simulink model "vnsimulink"  (R2020a)
settings: Solver=ode4  StartTime=0.0  StopTime=20  FixedStep=8e-6  RelTol=1e-3
undefined symbols (not defined in the file or in its folder): D1, Delta, sigbuilder_block
libraries: powerlib x98, powerlib_meascontrol x21, simulink x16
(part 2 of 3)

== system vnsimulink/PV15kW1/Subsystem2 ==
  Current : powerlib/Measurements/Current Measurement  PhasorSimulation=off  OutputType=Complex  PSBequivalent=0
  Current 2 : powerlib/Measurements/Current Measurement  PhasorSimulation=off  OutputType=Complex  PSBequivalent=0
  Current1 : powerlib/Measurements/Current Measurement  PhasorSimulation=off  OutputType=Complex  PSBequivalent=0
  1 : PMIOPort  Side=Left
  2 : PMIOPort  Port=2  Side=Right
  3 : PMIOPort  Port=3  Side=Left
  4 : PMIOPort  Port=4  Side=Right
  5 : PMIOPort  Port=5  Side=Left
  6 : PMIOPort  Port=6  Side=Right
  O1 : Outport
  O2 : Outport  Port=2
  O3 : Outport  Port=3
  wires:
  Current 2/1 -> O3/1
  Current1/1 -> O2/1
  Current/1 -> O1/1
  connections:
  6/RConn1 -- Current 2/RConn1
  5/RConn1 -- Current 2/LConn1
  4/RConn1 -- Current1/RConn1
  3/RConn1 -- Current1/LConn1
  2/RConn1 -- Current/RConn1
  1/RConn1 -- Current/LConn1

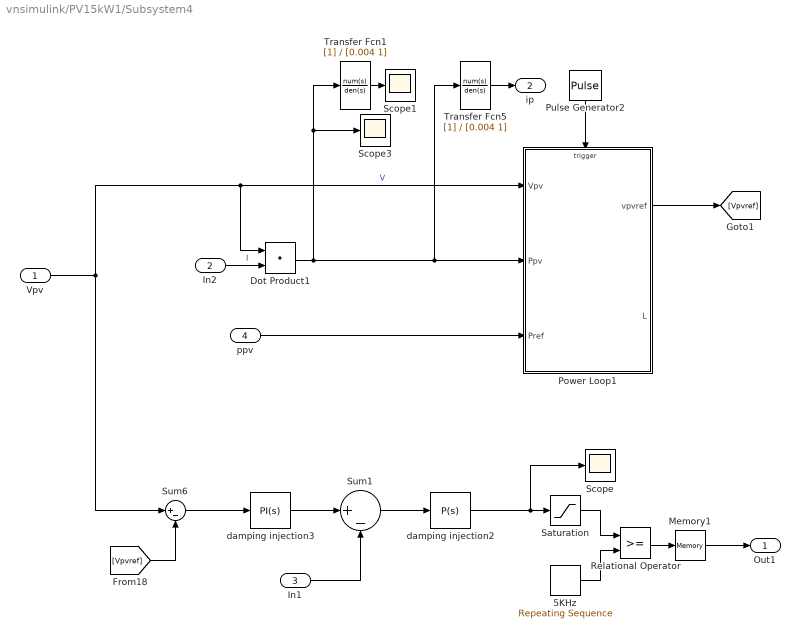
== system vnsimulink/PV15kW1/Subsystem4 ==
  Vpv : Inport
  In2 : Inport  Port=2
  In1 : Inport  Port=3
  ppv : Inport  Port=4
  5KHz : simulink/Sources/Repeating Sequence  rep_seq_t=[0 1e-4 2e-4]  rep_seq_y=[0 1 0]
  Dot Product1 : DotProduct  InputSameDT=on  OutDataTypeStr=Inherit: Inherit via internal rule
  Memory1 : Memory
  Power Loop1 : Subsystem  TreatAsAtomicUnit=on
  Pulse Generator2 : DiscretePulseGenerator  PulseType=Time based  Period=20e-4  PulseWidth=50
  Relational Operator : RelationalOperator  OutDataTypeStr=boolean  RndMeth=Nearest
  Saturation : Saturate  UpperLimit=0.9  LowerLimit=0
  Scope : Scope
  Scope1 : Scope
  Scope3 : Scope
  Sum1 : Sum  Inputs=|+-
  Sum6 : Sum  Inputs=|+-
  Transfer Fcn1 : TransferFcn  Denominator=[0.004 1]
  Transfer Fcn5 : TransferFcn  Denominator=[0.004 1]
  damping injection2 : simulink/Continuous/PID Controller  Controller=P  Form=Parallel  TimeDomain=Continuous-time  UseExternalTs=off  SampleTime=1  IntegratorMethod=Forward Euler  FilterMethod=Forward Euler  ControllerParametersSource=internal  P=0.015  I=0.15  D=0  UseFilter=on  N=100  TunerSelectOption=Transfer Function Based (PID Tuner App)  InitialConditionSource=internal  InitialConditionForIntegrator=0  InitialConditionForFilter=0  DifferentiatorICPrevScaledInput=0  ExternalReset=none  TrackingMode=off  Kt=1  LimitOutput=off  UpperSaturationLimit=inf  LowerSaturationLimit=-inf  LinearizeAsGain=on  AntiWindupMode=none  Kb=1  POutMin=[]  POutMax=[]  IOutMin=[]  IOutMax=[]  DOutMin=[]  DOutMax=[]  NOutMin=[]  NOutMax=[]  SumOutMin=[]  SumOutMax=[]  SaturationOutMin=[]  SaturationOutMax=[]  PParamMin=[]  PParamMax=[]  IParamMin=[]  IParamMax=[]  DParamMin=[]  DParamMax=[]  NParamMin=[]  NParamMax=[]  KbParamMin=[]  KbParamMax=[]  KtParamMin=[]  KtParamMax=[]  KbOutMin=[]  KbOutMax=[]  KtOutMin=[]  KtOutMax=[]  IntegratorOutMin=[]  IntegratorOutMax=[]  FilterOutMin=[]  FilterOutMax=[]  SumI1OutMin=[]  SumI1OutMax=[]  SumI2OutMin=[]  SumI2OutMax=[]  SumI3OutMin=[]  SumI3OutMax=[]  SumI4OutMin=[]  SumI4OutMax=[]  SumDOutMin=[]  SumDOutMax=[]  DifferentiatorOutMin=[]  DifferentiatorOutMax=[]  FilterDiffOutCoefMin=[]  FilterDiffOutCoefMax=[]  ReciprocalOutMin=[]  ReciprocalOutMax=[]  SumDenOutMin=[]  SumDenOutMax=[]  SumNumOutMin=[]  SumNumOutMax=[]  DivideOutMin=[]  DivideOutMax=[]  UdiffTsProdOutMin=[]  UdiffTsProdOutMax=[]  NTsProdOutMin=[]  NTsProdOutMax=[]  UintegralTsProdOutMin=[]  UintegralTsProdOutMax=[]  UngainTsProdOutMin=[]  UngainTsProdOutMax=[]  IntegratorContinuousStateAttributes=''  IntegratorStateMustResolveToSignalObject=off  IntegratorRTWStateStorageClass=Auto  FilterContinuousStateAttributes=''  FilterStateMustResolveToSignalObject=off  FilterRTWStateStorageClass=Auto  ParallelPVariant=InternalParameters  IdealPVariant=Disabled  IVariant=Disabled  DVariant=Disabled  IntegratorVariant=Disabled  SatVariant=Disabled  AWVariant=Disabled  PCopyVariant=Disabled  TRVariant=Disabled  FdbkBlocksVariant=Forward  IdealPFdbkVariant=Disabled  SatFdbkVariant=Disabled  DerivativeFilterVariant=Disabled  NVariant=Disabled  NCopyVariant=Disabled_SignalSpec  FilterICVariant=Disabled  IntegratorICVariant=Disabled  ExternalResetVariant=Disabled  TRSumVariant=Passthrough  SumFdbkVariant=Disabled  SumVariant=Passthrough_P  TsampFilterVariant=InternalTs  TsampNgainVariant=Passthrough  TsampIntegralVariant=Disabled_SignalSpec
  damping injection3 : simulink/Continuous/PID Controller  Controller=PI  Form=Parallel  TimeDomain=Continuous-time  UseExternalTs=off  SampleTime=1  IntegratorMethod=Forward Euler  FilterMethod=Forward Euler  ControllerParametersSource=internal  P=0.3  I=6  D=0  UseFilter=on  N=100  TunerSelectOption=Transfer Function Based (PID Tuner App)  InitialConditionSource=internal  InitialConditionForIntegrator=0  InitialConditionForFilter=0  DifferentiatorICPrevScaledInput=0  ExternalReset=none  TrackingMode=off  Kt=1  LimitOutput=off  UpperSaturationLimit=inf  LowerSaturationLimit=-inf  LinearizeAsGain=on  AntiWindupMode=none  Kb=1  POutMin=[]  POutMax=[]  IOutMin=[]  IOutMax=[]  DOutMin=[]  DOutMax=[]  NOutMin=[]  NOutMax=[]  SumOutMin=[]  SumOutMax=[]  SaturationOutMin=[]  SaturationOutMax=[]  PParamMin=[]  PParamMax=[]  IParamMin=[]  IParamMax=[]  DParamMin=[]  DParamMax=[]  NParamMin=[]  NParamMax=[]  KbParamMin=[]  KbParamMax=[]  KtParamMin=[]  KtParamMax=[]  KbOutMin=[]  KbOutMax=[]  KtOutMin=[]  KtOutMax=[]  IntegratorOutMin=[]  IntegratorOutMax=[]  FilterOutMin=[]  FilterOutMax=[]  SumI1OutMin=[]  SumI1OutMax=[]  SumI2OutMin=[]  SumI2OutMax=[]  SumI3OutMin=[]  SumI3OutMax=[]  SumI4OutMin=[]  SumI4OutMax=[]  SumDOutMin=[]  SumDOutMax=[]  DifferentiatorOutMin=[]  DifferentiatorOutMax=[]  FilterDiffOutCoefMin=[]  FilterDiffOutCoefMax=[]  ReciprocalOutMin=[]  ReciprocalOutMax=[]  SumDenOutMin=[]  SumDenOutMax=[]  SumNumOutMin=[]  SumNumOutMax=[]  DivideOutMin=[]  DivideOutMax=[]  UdiffTsProdOutMin=[]  UdiffTsProdOutMax=[]  NTsProdOutMin=[]  NTsProdOutMax=[]  UintegralTsProdOutMin=[]  UintegralTsProdOutMax=[]  UngainTsProdOutMin=[]  UngainTsProdOutMax=[]  IntegratorContinuousStateAttributes=''  IntegratorStateMustResolveToSignalObject=off  IntegratorRTWStateStorageClass=Auto  FilterContinuousStateAttributes=''  FilterStateMustResolveToSignalObject=off  FilterRTWStateStorageClass=Auto  ParallelPVariant=InternalParameters  IdealPVariant=Disabled  IVariant=InternalParameters  DVariant=Disabled  IntegratorVariant=Continuous  SatVariant=Disabled  AWVariant=Passthrough  PCopyVariant=Disabled  TRVariant=Disabled  FdbkBlocksVariant=Forward  IdealPFdbkVariant=Disabled  SatFdbkVariant=Disabled  DerivativeFilterVariant=Disabled  NVariant=Disabled  NCopyVariant=Disabled_SignalSpec  FilterICVariant=Disabled  IntegratorICVariant=InternalICs  ExternalResetVariant=Disabled  TRSumVariant=Passthrough  SumFdbkVariant=Disabled  SumVariant=Sum_PI  TsampFilterVariant=InternalTs  TsampNgainVariant=Passthrough  TsampIntegralVariant=Passthrough
  Out1 : Outport
  ip : Outport  Port=2
  wires:
  Transfer Fcn1/1 -> Scope1/1
  Transfer Fcn5/1 -> ip/1
  Dot Product1/1 -> Scope3/1, Transfer Fcn1/1, Power Loop1/2(Ppv), Transfer Fcn5/1
  Vpv/1 -> Sum6/1, Power Loop1/1(Vpv), Dot Product1/1  "V"
  In2/1 -> Dot Product1/2  "I"
  ppv/1 -> Power Loop1/3(Pref)
  Power Loop1/1(vpvref) -> [Vpvref]
  Pulse Generator2/1 -> Power Loop1/Trigger
  [Vpvref] -> Sum6/2
  Sum1/1 -> damping injection2/1
  Saturation/1 -> Relational Operator/1
  damping injection3/1 -> Sum1/1
  Relational Operator/1 -> Memory1/1
  Memory1/1 -> Out1/1
  damping injection2/1 -> Saturation/1, Scope/1
  5KHz/1 -> Relational Operator/2
  Sum6/1 -> damping injection3/1
  In1/1 -> Sum1/2

== system vnsimulink/PV15kW1/Subsystem7 ==
  Voltage : powerlib/Measurements/Voltage Measurement  PhasorSimulation=off  OutputType=Complex  PSBequivalent=0
  Voltage1 : powerlib/Measurements/Voltage Measurement  PhasorSimulation=off  OutputType=Complex  PSBequivalent=0
  Voltage2 : powerlib/Measurements/Voltage Measurement  PhasorSimulation=off  OutputType=Complex  PSBequivalent=0
  1 : PMIOPort  Side=Left
  2 : PMIOPort  Port=2  Side=Left
  3 : PMIOPort  Port=3  Side=Left
  4 : PMIOPort  Port=4  Side=Left
  5 : PMIOPort  Port=5  Side=Left
  6 : PMIOPort  Port=6  Side=Left
  O1 : Outport
  O2 : Outport  Port=2
  O3 : Outport  Port=3
  wires:
  Voltage/1 -> O1/1
  Voltage1/1 -> O2/1
  Voltage2/1 -> O3/1
  connections:
  1/RConn1 -- Voltage/LConn1
  2/RConn1 -- Voltage/LConn2
  3/RConn1 -- Voltage1/LConn1
  4/RConn1 -- Voltage1/LConn2
  5/RConn1 -- Voltage2/LConn1
  6/RConn1 -- Voltage2/LConn2

== system vnsimulink/PV15kW1/Subsystem8 ==
  Current : powerlib/Measurements/Current Measurement  PhasorSimulation=off  OutputType=Complex  PSBequivalent=0
  Current 2 : powerlib/Measurements/Current Measurement  PhasorSimulation=off  OutputType=Complex  PSBequivalent=0
  Current1 : powerlib/Measurements/Current Measurement  PhasorSimulation=off  OutputType=Complex  PSBequivalent=0
  1 : PMIOPort  Side=Left
  2 : PMIOPort  Port=2  Side=Right
  3 : PMIOPort  Port=3  Side=Left
  4 : PMIOPort  Port=4  Side=Right
  5 : PMIOPort  Port=5  Side=Left
  6 : PMIOPort  Port=6  Side=Right
  O1 : Outport
  O2 : Outport  Port=2
  O3 : Outport  Port=3
  wires:
  Current 2/1 -> O3/1
  Current1/1 -> O2/1
  Current/1 -> O1/1
  connections:
  6/RConn1 -- Current 2/RConn1
  5/RConn1 -- Current 2/LConn1
  4/RConn1 -- Current1/RConn1
  3/RConn1 -- Current1/LConn1
  2/RConn1 -- Current/RConn1
  1/RConn1 -- Current/LConn1

== system vnsimulink/PV15kW2/Irradiance Temp1 ==
  Demux : Demux  Tag=STV Demux  Outputs=1
      settings: DisplayOption=none
  FromWs : FromWorkspace  Tag=STV FromWs  VariableName=tuvar
      SigBuilderData=|
      | common.afterFinalStr = 'Extrapolate'
      | common.sampleTime = '0'
      | dataSet(1).timeRange = [0 7.5]
      | dataSet(1).name = 'Constant Irradiance'
      | dataSet(2).timeRange = [0 7.5]
      | dataSet(2).name = 'Step Irradiance'
      | dataSet(3).timeRange = [0 15]
      | dataSet(3).name = 'Ramp-up/down Irradiance'
      | sbobj.Groups(1).Name = 'Constant Irradiance'
      | sbobj.Groups(1).Signals.Name = 'Signal 2'
      | sbobj.Groups(1).Signals.XData = [0 3.75 3.75 7.5]
      | sbobj.Groups(1).Signals.YData = [0 0 1 1]
      | sbobj.Groups(1).TimeRange = [0 7.5]
      | sbobj.Groups(2).Name = 'Step Irradiance'
      | sbobj.Groups(2).Signals.Name = 'Signal 2'
      | sbobj.Groups(2).Signals.XData = [0 3.75 3.75 7.5]
      | sbobj.Groups(2).Signals.YData = [0 0 1 1]
      | sbobj.Groups(2).TimeRange = [0 7.5]
      | sbobj.Groups(3).Name = 'Ramp-up/down Irradiance'
      | sbobj.Groups(3).Signals.Name = 'Signal 2'
      | sbobj.Groups(3).Signals.XData = [0 10 12 15]
      | sbobj.Groups(3).Signals.YData = [1000 1000 900 900]
      | sbobj.Groups(3).TimeRange = [0 15]
  Signal 2 : Outport  Tag=STV Outport
  wires:
  Demux/1 -> Signal 2/1
  FromWs/1 -> Demux/1

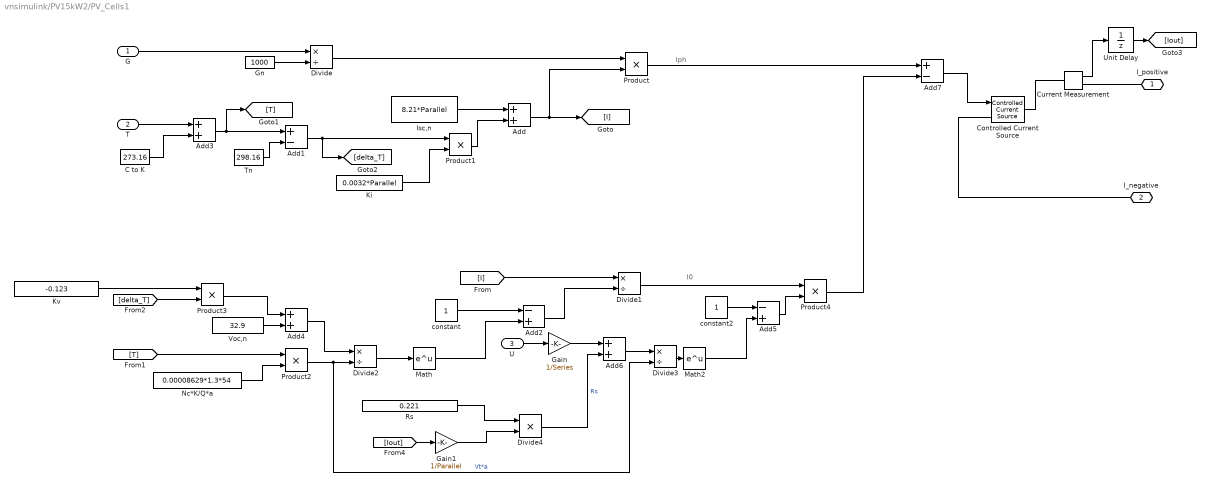
== system vnsimulink/PV15kW2/PV_Cells1 ==
  note: Iph
  note: I0
  G : Inport
  T : Inport  Port=2
  U : Inport  Port=3
  Add{,3..4,6} (4 alike) : Sum
  Add1 : Sum  Inputs=+-
  Add2 : Sum  Inputs=-+
  Add5 : Sum  Inputs=-+
  Add7 : Sum  Inputs=+-
  C to K : Constant  Value=273.16
  Controlled Current Source : powerlib/Electrical Sources/Controlled Current Source  Initialize=on  Source_Type=DC  Amplitude=0  Phase=0  Frequency=0  Measurements=None
  Current Measurement : powerlib/Measurements/Current Measurement  PhasorSimulation=off  OutputType=Complex  PSBequivalent=0
  Divide{,1..3} (4 alike) : Product  Inputs=*/
  Divide4 : Product  Inputs=**
  Gain : Gain  Gain=1/Series
  Gain1 : Gain  Gain=1/Parallel
  Gn : Constant  Value=1000
  Isc,n : Constant  Value=8.21*Parallel
  Ki : Constant  Value=0.0032*Parallel
  Kv : Constant  Value=-0.123
  Math : Math  SignedPower=on  SaturateOnIntegerOverflow=on
  Math2 : Math  SignedPower=on  SaturateOnIntegerOverflow=on
  Nc*K/Q*a : Constant  Value=0.00008629*1.3*54
  Product{,1..4} (5 alike) : Product  RndMeth=Zero
  Rs : Constant  Value=0.221
  Tn : Constant  Value=298.16
  Unit Delay : UnitDelay  SampleTime=-1  HasFrameUpgradeWarning=on
  Voc,n : Constant  Value=32.9
  constant : Constant
  constant2 : Constant
  I_positive : PMIOPort  Tag=PMCPort  Side=Right
  I_negative : PMIOPort  Tag=PMCPort  Port=2  Side=Right
  wires:
  Divide4/1 -> Add6/2  "Rs"
  Gain1/1 -> Divide4/2
  Gain/1 -> Add6/1
  Unit Delay/1 -> [Iout]
  G/1 -> Divide/1
  Add3/1 -> Add1/1, [T]
  constant/1 -> Add2/1
  Gn/1 -> Divide/2
  Product3/1 -> Add4/1
  Add4/1 -> Divide2/1
  Product2/1 -> Divide2/2, Divide3/2  "Vt*a"
  C to K/1 -> Add3/2
  Divide3/1 -> Math2/1
  Math2/1 -> Add5/2
  [Iout] -> Gain1/1
  Add5/1 -> Product4/2
  constant2/1 -> Add5/1
  Product4/1 -> Add7/2
  Add7/1 -> Controlled Current Source/1
  Divide1/1 -> Product4/1
  Rs/1 -> Divide4/1
  U/1 -> Gain/1
  Add6/1 -> Divide3/1
  [delta_T] -> Product3/2
  [T] -> Product2/1
  Current Measurement/1 -> Unit Delay/1
  Voc,n/1 -> Add4/2
  Kv/1 -> Product3/1
  Nc*K/Q*a/1 -> Product2/2
  Product/1 -> Add7/1
  Ki/1 -> Product1/2
  Tn/1 -> Add1/2
  Add1/1 -> Product1/1, [delta_T]
  [I] -> Divide1/1
  Math/1 -> Add2/2
  Add2/1 -> Divide1/2
  T/1 -> Add3/1
  Add/1 -> Product/2, [I]
  Divide2/1 -> Math/1
  Product1/1 -> Add/2
  Isc,n/1 -> Add/1
  Divide/1 -> Product/1
  connections:
  Controlled Current Source/RConn1 -- Current Measurement/LConn1
  I_positive/RConn1 -- Current Measurement/RConn1
  I_negative/RConn1 -- Controlled Current Source/LConn1

== system vnsimulink/PV15kW2/PWM2 ==
  Via* : Inport
  Vib* : Inport  Port=2
  Vi0* : Inport  Port=3
  Alpha-Beta-Zero to abc1 : powerlib_meascontrol/Transformations/Alpha-Beta-Zero to abc
      settings: SourceProductBaseCode=PS
  Bus Creator : BusCreator  Inputs=3
  Demux : Demux  Outputs=3
  Mux1 : Mux  Inputs=3
  PWM : Subsystem
  Scope : Scope
  Transport Delay2 : TransportDelay  DelayTime=2e-4
  switch : Outport  PortDimensions=6
  Out1 : Outport  Port=2
  wires:
  PWM/2(Out1) -> Out1/1
  Bus Creator/1 -> Scope/1, PWM/1(In1)
  Via*/1 -> Mux1/1
  Vib*/1 -> Mux1/2
  Vi0*/1 -> Mux1/3
  Demux/2 -> Bus Creator/2
  Demux/3 -> Bus Creator/3
  PWM/1(switch) -> switch/1
  Demux/1 -> Bus Creator/1
  Alpha-Beta-Zero to abc1/1 -> Demux/1
  Mux1/1 -> Transport Delay2/1
  Transport Delay2/1 -> Alpha-Beta-Zero to abc1/1

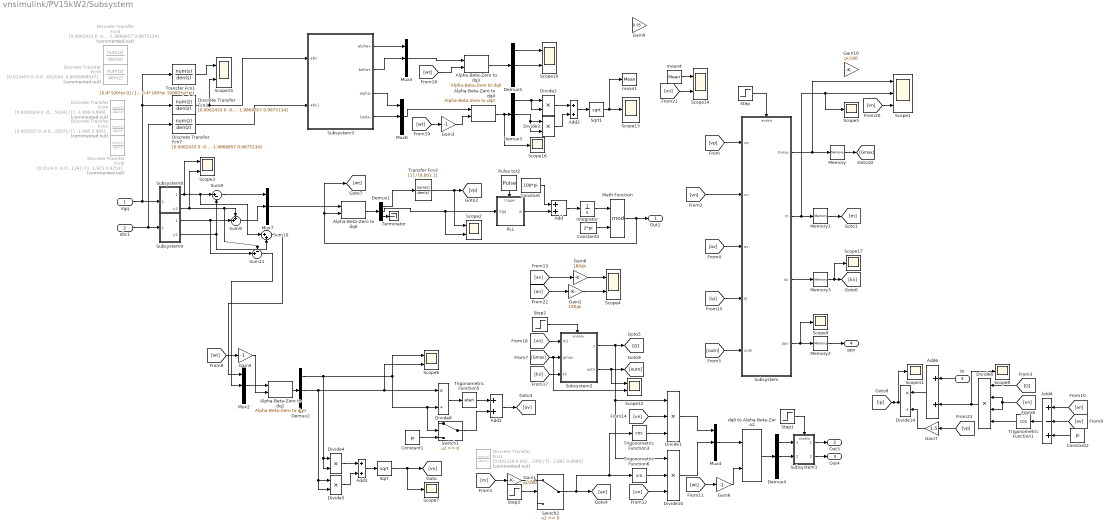
== system vnsimulink/PV15kW2/Subsystem ==
  Vgq : Inport
  abc1 : Inport  Port=2
  ip : Inport  Port=3
  Add{,1..3,6} (5 alike) : Sum
  Add4 : Sum  Inputs=+-+
  Alpha-Beta-Zero to dq{0..1,3..4} (4 alike) : powerlib_meascontrol/Transformations/Alpha-Beta-Zero to dq0  Alignment=Aligned with phase A axis
  Constant : Constant  Value=100*pi
  Constant1 : Constant  Value=pi
  Constant2 : Constant  Value=pi
  Constant4 : Constant  Value=2*pi
  Demux{1..5} (5 alike) : Demux  Outputs=3
  Discrete Transfer Fcn1 : DiscreteTransferFcn  Commented=on  Numerator=[0.001339 0.002677 0.001339]  Denominator=[1 -1.881 0.8864]  SampleTime=2e-4
  Discrete Transfer Fcn2 : DiscreteTransferFcn  Commented=on  Numerator=[0.002507 0 -0.002507]  Denominator=[1 -1.995 0.995]  SampleTime=4e-5
  Discrete Transfer Fcn3 : DiscreteTransferFcn  Numerator=[0.0062433 0 -0.0062433]  Denominator=[1 -1.9868857 0.9875134]  SampleTime=8e-5
  Discrete Transfer Fcn4 : DiscreteTransferFcn  Commented=on  Numerator=[0.0005024 0 -0.0005024]  Denominator=[1 -1.999 0.999]
  Discrete Transfer Fcn5 : DiscreteTransferFcn  Commented=on  Numerator=[0.0062433 0 -0.0062433]  Denominator=[1 -1.9868857 0.9875134]  SampleTime=8e-5
  Discrete Transfer Fcn6 : DiscreteTransferFcn  Commented=on  Numerator=[0.0124 0 -0.0124]  Denominator=[1 -1.971 0.9752]  SampleTime=2e-4
  Discrete Transfer Fcn7 : DiscreteTransferFcn  Numerator=[0.0062433 0 -0.0062433]  Denominator=[1 -1.9868857 0.9875134]  SampleTime=8e-5
  Discrete Transfer Fcn8 : DiscreteTransferFcn  Commented=on  Numerator=[0.015455 0 -0.015455]  Denominator="[1 -1.9652044  0.9690899547]"  SampleTime=2e-4
  Divide1 : Product  Inputs=***
  Divide10 : Product  Inputs=***
  Divide14 : Product  Inputs=*/
  Divide{2..5} (4 alike) : Product  Inputs=**
  Divide6 : Product  Inputs=****
  Divide8 : Product  Inputs=*/
  Gain1 : Gain  Gain=pi/180
  Gain10 : Gain  Gain=pi/180
  Gain2 : Gain  Gain=180/pi
  Gain3 : Gain  Gain=-1
  Gain5 : Gain  Gain=-1
  Gain6 : Gain  Gain=-1
  Gain7 : Gain  Gain=1.5
  Gain8 : Gain  Gain=180/pi
  Gain9 : Gain  Gain=0.95
  Integrator : Integrator
  Math Function : Math  Operator=mod  SignedPower=on  SaturateOnIntegerOverflow=on
  Memory{,1..3} (4 alike) : Memory
  Mux{2,4..7} (5 alike) : Mux  Inputs=3
  PLL : Subsystem  TreatAsAtomicUnit=on
  Pulse tor2 : DiscretePulseGenerator  PulseType=Time based  Period=2e-4  PulseWidth=40
  Scope1 : Scope  NumInputPorts=3
  Scope{2..4,6,10,12,14..15} (8 alike) : Scope  NumInputPorts=2
  Scope{5,7..9,11,13,16..17} (8 alike) : Scope
  Sqrt : Sqrt  SaturateOnIntegerOverflow=on
  Sqrt1 : Sqrt  SaturateOnIntegerOverflow=on
  Step : Step  Time=0.9922  SampleTime=0
  Step1 : Step  SampleTime=0
  Step2 : Step  SampleTime=0
  Step3 : Step  SampleTime=0
  Subsystem : Subsystem
  Subsystem1 : Subsystem
  Subsystem2 : Subsystem
  Subsystem3 : Subsystem
  Subsystem8 : Subsystem
  Subsystem9 : Subsystem
  Sum10 : Sum  Inputs=|++
  Sum11 : Sum  Inputs=-+|
  Sum8 : Sum  Inputs=|+-
  Sum9 : Sum  Inputs=++|
  Switch1 : Switch
  Switch2 : Switch
  Terminator : Terminator
  Transfer Fcn1 : TransferFcn  Numerator=[0.4*100*pi 0]  Denominator=[1 0.4*100*pi 10000*pi*pi]
  Transfer Fcn3 : TransferFcn  Denominator=[0.001 1]
  Trigonometric Function1 : Trigonometry  Operator=cos
  Trigonometric Function3 : Trigonometry  Operator=cos
  Trigonometric Function5 : Trigonometry  Operator=atan
  Trigonometric Function6 : Trigonometry
  dq0 to Alpha-Beta-Zero2 : powerlib_meascontrol/Transformations/dq0 to Alpha-Beta-Zero  Alignment=Aligned with phase A axis
      settings: SourceProductBaseCode=PS
  mean1 : powerlib_meascontrol/Measurements/Mean  Freq=50  Vinit=0  Ts=20e-5
  mean4 : powerlib_meascontrol/Measurements/Mean  Freq=50  Vinit=0  Ts=20e-5
  Out1 : Outport
  Out3 : Outport  Port=2
  Out4 : Outport  Port=3
  ppv : Outport  Port=4
  wires:
  Add/1 -> Integrator/1
  Math Function/1 -> Out1/1, [wt], Alpha-Beta-Zero to dq0/2
  Constant/1 -> Add/1
  PLL/1(w) -> Add/2
  Alpha-Beta-Zero to dq0/1 -> Demux1/1
  Demux1/1 -> Transfer Fcn3/1
  Constant4/1 -> Math Function/2
  Pulse tor2/1 -> PLL/Trigger
  Integrator/1 -> Math Function/1
  Mux2/1 -> Alpha-Beta-Zero to dq1/1
  Alpha-Beta-Zero to dq1/1 -> Demux2/1
  Constant1/1 -> Switch1/3
  Divide8/1 -> Trigonometric Function5/1
  Add3/1 -> Sqrt/1
  Divide4/1 -> Add3/1
  Divide5/1 -> Add3/2
  [wt] -> Gain5/1
  Divide10/1 -> Mux4/2
  [wt] -> Gain6/1
  Trigonometric Function3/1 -> Divide1/3
  [vn] -> Divide10/3
  Step/1 -> Subsystem/Enable
  Divide1/1 -> Mux4/1
  Mux4/1 -> dq0 to Alpha-Beta-Zero2/1
  Demux4/1 -> Subsystem1/1(In2)
  Demux4/2 -> Subsystem1/2(In3)
  Step1/1 -> Subsystem1/Enable
  Subsystem1/2(Out4) -> Out4/1
  Gain5/1 -> Alpha-Beta-Zero to dq1/2
  Gain6/1 -> dq0 to Alpha-Beta-Zero2/2
  Subsystem/1(Gmax) -> Scope1/1, Memory/1
  [vn] -> Subsystem2/1(In1)
  Step2/1 -> Subsystem2/Enable
  Subsystem/4(ppv) -> Memory2/1, Scope9/1
  Subsystem2/2(outn) -> Scope12/1, [outn]
  Memory/1 -> [Gmax]
  Gain8/1 -> Scope4/1
  Gain2/1 -> Scope4/2
  Trigonometric Function5/1 -> Add1/1
  Add1/1 -> [av]
  Switch1/1 -> Add1/2
  [vp] -> Gain7/1
  [av] -> Subsystem/3(av)
  Transfer Fcn3/1 -> Scope2/1, [vp]
  ip/1 -> Add6/1
  Add6/1 -> Divide14/1
  Gain7/1 -> Divide14/2
  Memory2/1 -> ppv/1
  Subsystem8/1(Out1) -> Scope3/1, Sum10/1, Sum8/1
  Subsystem9/2(y2) -> Sum8/2, Sum10/2
  Subsystem9/1(Out1) -> Sum11/2, Sum9/2
  Subsystem8/2(y2) -> Scope3/2, Sum11/1, Sum9/1
  Sum8/1 -> Mux7/1
  Sum9/1 -> Mux7/2
  dq0 to Alpha-Beta-Zero2/1 -> Demux4/1
  Subsystem1/1(Out3) -> Out3/1
  Subsystem2/1(y) -> [G], Divide1/1, Divide10/1
  Trigonometric Function6/1 -> Divide10/2
  [an] -> Gain2/1
  Step3/1 -> Switch2/2
  Gain1/1 -> Switch2/1
  Memory1/1 -> [m]
  Subsystem/2(m) -> Memory1/1, Scope1/2, Scope5/1
  [m] -> Gain1/1
  [vp] -> Subsystem/1(vp)
  Demux1/3 -> Terminator/1
  [outn] -> Subsystem/5(outn)
  [Gmax] -> Scope12/2, Subsystem2/2(gmax)
  Switch2/1 -> [an], Trigonometric Function6/1, Trigonometric Function3/1
  Add4/1 -> Trigonometric Function1/1
  [vn] -> Divide6/3, Divide6/2
  Trigonometric Function1/1 -> Divide6/4
  [av] -> Add4/2
  [an] -> Add4/1
  [G] -> Divide6/1
  Divide6/1 -> Add6/2, Scope8/1
  [av] -> Gain8/1
  Constant2/1 -> Add4/3
  [ip] -> Subsystem/4(ip)
  Divide14/1 -> Scope11/1, [ip]
  [kii] -> Subsystem2/3(kii)
  Memory3/1 -> Scope17/1, [kii]
  [vn] -> Divide1/2
  Subsystem/3(kii) -> Memory3/1
  [vn] -> Scope1/3
  Demux2/1 -> Divide4/2, Divide4/1, Scope6/1, Switch1/2, Divide8/2
  Demux2/2 -> Divide5/2, Divide5/1, Scope6/2, Divide8/1
  Sum10/1 -> Mux2/1
  Sum11/1 -> Mux2/2
  Vgq/1 -> Discrete Transfer Fcn3/1, Transfer Fcn1/1, Subsystem8/1(Vgq)
  abc1/1 -> Discrete Transfer Fcn7/1, Subsystem9/1(Vgq)
  [wt] -> Gain3/1
  [wt] -> Alpha-Beta-Zero to dq3/2
  Subsystem3/3(alpha-) -> Mux6/1
  Mux6/1 -> Alpha-Beta-Zero to dq4/1
  Subsystem3/1(alpha+) -> Mux5/1
  Gain3/1 -> Alpha-Beta-Zero to dq4/2
  Subsystem3/2(belta+) -> Mux5/2
  Subsystem3/4(belta-) -> Mux6/2
  Mux5/1 -> Alpha-Beta-Zero to dq3/1
  Alpha-Beta-Zero to dq3/1 -> Demux5/1
  Alpha-Beta-Zero to dq4/1 -> Scope16/1, Demux3/1
  Demux3/1 -> Divide2/1, Divide2/2
  Add2/1 -> Sqrt1/1
  Demux3/2 -> Divide3/2, Divide3/1
  Divide3/1 -> Add2/2
  Divide2/1 -> Add2/1
  mean4/1 -> Scope14/1
  [vn] -> Scope14/2
  Transfer Fcn1/1 -> Scope15/1
  Discrete Transfer Fcn7/1 -> Subsystem3/2(abc1)
  Discrete Transfer Fcn3/1 -> Scope15/2, Subsystem3/1(abc)
  Sqrt1/1 -> mean1/1, Scope13/1
  Demux5/1 -> Scope10/1
  Demux5/2 -> Scope10/2
  Demux1/2 -> Scope2/2, PLL/1(Vgq)
  Mux7/1 -> Alpha-Beta-Zero to dq0/1
  Sqrt/1 -> Scope7/1, [vn]
  [vn] -> Subsystem/2(vn)

== system vnsimulink/PV15kW2/Subsystem10 ==
  Current : powerlib/Measurements/Current Measurement  PhasorSimulation=off  OutputType=Complex  PSBequivalent=0
  Current 2 : powerlib/Measurements/Current Measurement  PhasorSimulation=off  OutputType=Complex  PSBequivalent=0
  Current1 : powerlib/Measurements/Current Measurement  PhasorSimulation=off  OutputType=Complex  PSBequivalent=0
  1 : PMIOPort  Side=Left
  2 : PMIOPort  Port=2  Side=Right
  3 : PMIOPort  Port=3  Side=Left
  4 : PMIOPort  Port=4  Side=Right
  5 : PMIOPort  Port=5  Side=Left
  6 : PMIOPort  Port=6  Side=Right
  O1 : Outport
  O2 : Outport  Port=2
  O3 : Outport  Port=3
  wires:
  Current/1 -> O1/1
  Current1/1 -> O2/1
  Current 2/1 -> O3/1
  connections:
  1/RConn1 -- Current/LConn1
  2/RConn1 -- Current/RConn1
  3/RConn1 -- Current1/LConn1
  4/RConn1 -- Current1/RConn1
  5/RConn1 -- Current 2/LConn1
  6/RConn1 -- Current 2/RConn1

== system vnsimulink/PV15kW2/Subsystem2 ==
  Current : powerlib/Measurements/Current Measurement  PhasorSimulation=off  OutputType=Complex  PSBequivalent=0
  Current 2 : powerlib/Measurements/Current Measurement  PhasorSimulation=off  OutputType=Complex  PSBequivalent=0
  Current1 : powerlib/Measurements/Current Measurement  PhasorSimulation=off  OutputType=Complex  PSBequivalent=0
  1 : PMIOPort  Side=Left
  2 : PMIOPort  Port=2  Side=Right
  3 : PMIOPort  Port=3  Side=Left
  4 : PMIOPort  Port=4  Side=Right
  5 : PMIOPort  Port=5  Side=Left
  6 : PMIOPort  Port=6  Side=Right
  O1 : Outport
  O2 : Outport  Port=2
  O3 : Outport  Port=3
  wires:
  Current/1 -> O1/1
  Current1/1 -> O2/1
  Current 2/1 -> O3/1
  connections:
  1/RConn1 -- Current/LConn1
  2/RConn1 -- Current/RConn1
  3/RConn1 -- Current1/LConn1
  4/RConn1 -- Current1/RConn1
  5/RConn1 -- Current 2/LConn1
  6/RConn1 -- Current 2/RConn1

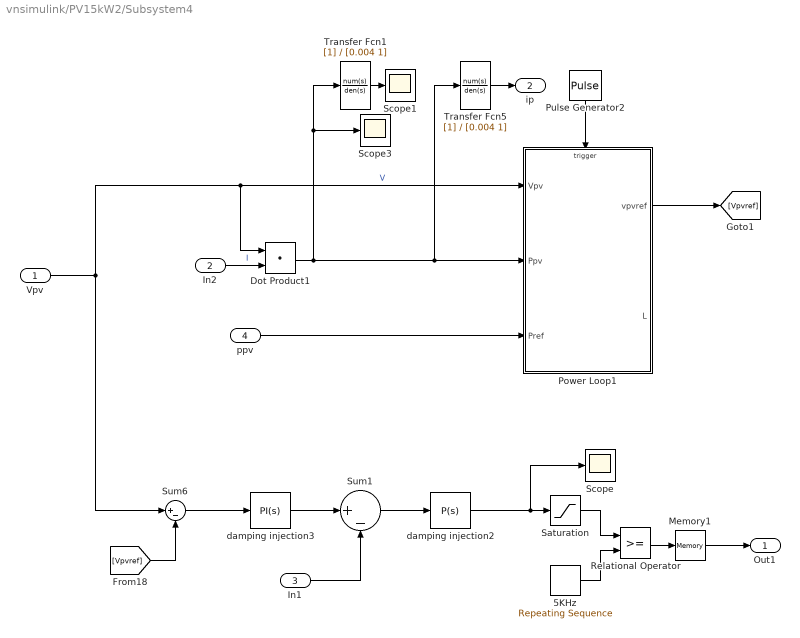
== system vnsimulink/PV15kW2/Subsystem4 ==
  Vpv : Inport
  In2 : Inport  Port=2
  In1 : Inport  Port=3
  ppv : Inport  Port=4
  5KHz : simulink/Sources/Repeating Sequence  rep_seq_t=[0 1e-4 2e-4]  rep_seq_y=[0 1 0]
  Dot Product1 : DotProduct  InputSameDT=on  OutDataTypeStr=Inherit: Inherit via internal rule
  Memory1 : Memory
  Power Loop1 : Subsystem  TreatAsAtomicUnit=on
  Pulse Generator2 : DiscretePulseGenerator  PulseType=Time based  Period=20e-4  PulseWidth=50
  Relational Operator : RelationalOperator  OutDataTypeStr=boolean  RndMeth=Nearest
  Saturation : Saturate  UpperLimit=0.9  LowerLimit=0
  Scope : Scope
  Scope1 : Scope
  Scope3 : Scope
  Sum1 : Sum  Inputs=|+-
  Sum6 : Sum  Inputs=|+-
  Transfer Fcn1 : TransferFcn  Denominator=[0.004 1]
  Transfer Fcn5 : TransferFcn  Denominator=[0.004 1]
  damping injection2 : simulink/Continuous/PID Controller  Controller=P  Form=Parallel  TimeDomain=Continuous-time  UseExternalTs=off  SampleTime=1  IntegratorMethod=Forward Euler  FilterMethod=Forward Euler  ControllerParametersSource=internal  P=0.015  I=0.15  D=0  UseFilter=on  N=100  TunerSelectOption=Transfer Function Based (PID Tuner App)  InitialConditionSource=internal  InitialConditionForIntegrator=0  InitialConditionForFilter=0  DifferentiatorICPrevScaledInput=0  ExternalReset=none  TrackingMode=off  Kt=1  LimitOutput=off  UpperSaturationLimit=inf  LowerSaturationLimit=-inf  LinearizeAsGain=on  AntiWindupMode=none  Kb=1  POutMin=[]  POutMax=[]  IOutMin=[]  IOutMax=[]  DOutMin=[]  DOutMax=[]  NOutMin=[]  NOutMax=[]  SumOutMin=[]  SumOutMax=[]  SaturationOutMin=[]  SaturationOutMax=[]  PParamMin=[]  PParamMax=[]  IParamMin=[]  IParamMax=[]  DParamMin=[]  DParamMax=[]  NParamMin=[]  NParamMax=[]  KbParamMin=[]  KbParamMax=[]  KtParamMin=[]  KtParamMax=[]  KbOutMin=[]  KbOutMax=[]  KtOutMin=[]  KtOutMax=[]  IntegratorOutMin=[]  IntegratorOutMax=[]  FilterOutMin=[]  FilterOutMax=[]  SumI1OutMin=[]  SumI1OutMax=[]  SumI2OutMin=[]  SumI2OutMax=[]  SumI3OutMin=[]  SumI3OutMax=[]  SumI4OutMin=[]  SumI4OutMax=[]  SumDOutMin=[]  SumDOutMax=[]  DifferentiatorOutMin=[]  DifferentiatorOutMax=[]  FilterDiffOutCoefMin=[]  FilterDiffOutCoefMax=[]  ReciprocalOutMin=[]  ReciprocalOutMax=[]  SumDenOutMin=[]  SumDenOutMax=[]  SumNumOutMin=[]  SumNumOutMax=[]  DivideOutMin=[]  DivideOutMax=[]  UdiffTsProdOutMin=[]  UdiffTsProdOutMax=[]  NTsProdOutMin=[]  NTsProdOutMax=[]  UintegralTsProdOutMin=[]  UintegralTsProdOutMax=[]  UngainTsProdOutMin=[]  UngainTsProdOutMax=[]  IntegratorContinuousStateAttributes=''  IntegratorStateMustResolveToSignalObject=off  IntegratorRTWStateStorageClass=Auto  FilterContinuousStateAttributes=''  FilterStateMustResolveToSignalObject=off  FilterRTWStateStorageClass=Auto  ParallelPVariant=InternalParameters  IdealPVariant=Disabled  IVariant=Disabled  DVariant=Disabled  IntegratorVariant=Disabled  SatVariant=Disabled  AWVariant=Disabled  PCopyVariant=Disabled  TRVariant=Disabled  FdbkBlocksVariant=Forward  IdealPFdbkVariant=Disabled  SatFdbkVariant=Disabled  DerivativeFilterVariant=Disabled  NVariant=Disabled  NCopyVariant=Disabled_SignalSpec  FilterICVariant=Disabled  IntegratorICVariant=Disabled  ExternalResetVariant=Disabled  TRSumVariant=Passthrough  SumFdbkVariant=Disabled  SumVariant=Passthrough_P  TsampFilterVariant=InternalTs  TsampNgainVariant=Passthrough  TsampIntegralVariant=Disabled_SignalSpec
  damping injection3 : simulink/Continuous/PID Controller  Controller=PI  Form=Parallel  TimeDomain=Continuous-time  UseExternalTs=off  SampleTime=1  IntegratorMethod=Forward Euler  FilterMethod=Forward Euler  ControllerParametersSource=internal  P=0.3  I=6  D=0  UseFilter=on  N=100  TunerSelectOption=Transfer Function Based (PID Tuner App)  InitialConditionSource=internal  InitialConditionForIntegrator=0  InitialConditionForFilter=0  DifferentiatorICPrevScaledInput=0  ExternalReset=none  TrackingMode=off  Kt=1  LimitOutput=off  UpperSaturationLimit=inf  LowerSaturationLimit=-inf  LinearizeAsGain=on  AntiWindupMode=none  Kb=1  POutMin=[]  POutMax=[]  IOutMin=[]  IOutMax=[]  DOutMin=[]  DOutMax=[]  NOutMin=[]  NOutMax=[]  SumOutMin=[]  SumOutMax=[]  SaturationOutMin=[]  SaturationOutMax=[]  PParamMin=[]  PParamMax=[]  IParamMin=[]  IParamMax=[]  DParamMin=[]  DParamMax=[]  NParamMin=[]  NParamMax=[]  KbParamMin=[]  KbParamMax=[]  KtParamMin=[]  KtParamMax=[]  KbOutMin=[]  KbOutMax=[]  KtOutMin=[]  KtOutMax=[]  IntegratorOutMin=[]  IntegratorOutMax=[]  FilterOutMin=[]  FilterOutMax=[]  SumI1OutMin=[]  SumI1OutMax=[]  SumI2OutMin=[]  SumI2OutMax=[]  SumI3OutMin=[]  SumI3OutMax=[]  SumI4OutMin=[]  SumI4OutMax=[]  SumDOutMin=[]  SumDOutMax=[]  DifferentiatorOutMin=[]  DifferentiatorOutMax=[]  FilterDiffOutCoefMin=[]  FilterDiffOutCoefMax=[]  ReciprocalOutMin=[]  ReciprocalOutMax=[]  SumDenOutMin=[]  SumDenOutMax=[]  SumNumOutMin=[]  SumNumOutMax=[]  DivideOutMin=[]  DivideOutMax=[]  UdiffTsProdOutMin=[]  UdiffTsProdOutMax=[]  NTsProdOutMin=[]  NTsProdOutMax=[]  UintegralTsProdOutMin=[]  UintegralTsProdOutMax=[]  UngainTsProdOutMin=[]  UngainTsProdOutMax=[]  IntegratorContinuousStateAttributes=''  IntegratorStateMustResolveToSignalObject=off  IntegratorRTWStateStorageClass=Auto  FilterContinuousStateAttributes=''  FilterStateMustResolveToSignalObject=off  FilterRTWStateStorageClass=Auto  ParallelPVariant=InternalParameters  IdealPVariant=Disabled  IVariant=InternalParameters  DVariant=Disabled  IntegratorVariant=Continuous  SatVariant=Disabled  AWVariant=Passthrough  PCopyVariant=Disabled  TRVariant=Disabled  FdbkBlocksVariant=Forward  IdealPFdbkVariant=Disabled  SatFdbkVariant=Disabled  DerivativeFilterVariant=Disabled  NVariant=Disabled  NCopyVariant=Disabled_SignalSpec  FilterICVariant=Disabled  IntegratorICVariant=InternalICs  ExternalResetVariant=Disabled  TRSumVariant=Passthrough  SumFdbkVariant=Disabled  SumVariant=Sum_PI  TsampFilterVariant=InternalTs  TsampNgainVariant=Passthrough  TsampIntegralVariant=Passthrough
  Out1 : Outport
  ip : Outport  Port=2
  wires:
  In1/1 -> Sum1/2
  Sum6/1 -> damping injection3/1
  5KHz/1 -> Relational Operator/2
  damping injection2/1 -> Scope/1, Saturation/1
  Memory1/1 -> Out1/1
  Relational Operator/1 -> Memory1/1
  damping injection3/1 -> Sum1/1
  Saturation/1 -> Relational Operator/1
  Sum1/1 -> damping injection2/1
  [Vpvref] -> Sum6/2
  Pulse Generator2/1 -> Power Loop1/Trigger
  Power Loop1/1(vpvref) -> [Vpvref]
  ppv/1 -> Power Loop1/3(Pref)
  In2/1 -> Dot Product1/2  "I"
  Vpv/1 -> Dot Product1/1, Power Loop1/1(Vpv), Sum6/1  "V"
  Dot Product1/1 -> Transfer Fcn5/1, Power Loop1/2(Ppv), Transfer Fcn1/1, Scope3/1
  Transfer Fcn5/1 -> ip/1
  Transfer Fcn1/1 -> Scope1/1

== system vnsimulink/PV15kW2/Subsystem7 ==
  Voltage : powerlib/Measurements/Voltage Measurement  PhasorSimulation=off  OutputType=Complex  PSBequivalent=0
  Voltage1 : powerlib/Measurements/Voltage Measurement  PhasorSimulation=off  OutputType=Complex  PSBequivalent=0
  Voltage2 : powerlib/Measurements/Voltage Measurement  PhasorSimulation=off  OutputType=Complex  PSBequivalent=0
  1 : PMIOPort  Side=Left
  2 : PMIOPort  Port=2  Side=Left
  3 : PMIOPort  Port=3  Side=Left
  4 : PMIOPort  Port=4  Side=Left
  5 : PMIOPort  Port=5  Side=Left
  6 : PMIOPort  Port=6  Side=Left
  O1 : Outport
  O2 : Outport  Port=2
  O3 : Outport  Port=3
  wires:
  Voltage2/1 -> O3/1
  Voltage1/1 -> O2/1
  Voltage/1 -> O1/1
  connections:
  6/RConn1 -- Voltage2/LConn2
  5/RConn1 -- Voltage2/LConn1
  4/RConn1 -- Voltage1/LConn2
  3/RConn1 -- Voltage1/LConn1
  2/RConn1 -- Voltage/LConn2
  1/RConn1 -- Voltage/LConn1

== system vnsimulink/PV15kW2/Subsystem8 ==
  Current : powerlib/Measurements/Current Measurement  PhasorSimulation=off  OutputType=Complex  PSBequivalent=0
  Current 2 : powerlib/Measurements/Current Measurement  PhasorSimulation=off  OutputType=Complex  PSBequivalent=0
  Current1 : powerlib/Measurements/Current Measurement  PhasorSimulation=off  OutputType=Complex  PSBequivalent=0
  1 : PMIOPort  Side=Left
  2 : PMIOPort  Port=2  Side=Right
  3 : PMIOPort  Port=3  Side=Left
  4 : PMIOPort  Port=4  Side=Right
  5 : PMIOPort  Port=5  Side=Left
  6 : PMIOPort  Port=6  Side=Right
  O1 : Outport
  O2 : Outport  Port=2
  O3 : Outport  Port=3
  wires:
  Current/1 -> O1/1
  Current1/1 -> O2/1
  Current 2/1 -> O3/1
  connections:
  1/RConn1 -- Current/LConn1
  2/RConn1 -- Current/RConn1
  3/RConn1 -- Current1/LConn1
  4/RConn1 -- Current1/RConn1
  5/RConn1 -- Current 2/LConn1
  6/RConn1 -- Current 2/RConn1

== system vnsimulink/PV15kW1/PWM2/PWM ==
  In1 : Inport
  Bus Creator1 : BusCreator  Inputs=6
  Constant : Constant
  Demux1 : Demux  Outputs=3
  Gain : Gain  Gain=1/1
  Logical Operator : Logic  Operator=NOT  AllPortsSameDT=off  OutDataTypeStr=boolean
  Logical Operator1 : Logic  Operator=NOT  AllPortsSameDT=off  OutDataTypeStr=boolean
  Logical Operator2 : Logic  Operator=NOT  AllPortsSameDT=off  OutDataTypeStr=boolean
  Relational Operator : RelationalOperator  OutDataTypeStr=boolean  RndMeth=Nearest
  Relational Operator1 : RelationalOperator  OutDataTypeStr=boolean  RndMeth=Nearest
  Relational Operator2 : RelationalOperator  OutDataTypeStr=boolean  RndMeth=Nearest
  Repeating Sequence : simulink/Sources/Repeating Sequence  rep_seq_t=[0 1e-4 2e-4]  rep_seq_y=[0 2 0]
  Sum : Sum  Inputs=|++
  switch : Outport  PortDimensions=6
  Out1 : Outport  Port=2
  wires:
  In1/1 -> Gain/1
  Logical Operator2/1 -> Bus Creator1/6
  Relational Operator2/1 -> Logical Operator2/1, Bus Creator1/5
  Demux1/3 -> Relational Operator2/1
  Logical Operator1/1 -> Bus Creator1/4
  Relational Operator1/1 -> Logical Operator1/1, Bus Creator1/3
  Demux1/2 -> Relational Operator1/1
  Logical Operator/1 -> Bus Creator1/2
  Relational Operator/1 -> Logical Operator/1, Bus Creator1/1
  Demux1/1 -> Relational Operator/1
  Sum/1 -> Out1/1, Demux1/1
  Gain/1 -> Sum/2
  Constant/1 -> Sum/1
  Repeating Sequence/1 -> Relational Operator2/2, Relational Operator1/2, Relational Operator/2
  Bus Creator1/1 -> switch/1

== system vnsimulink/PV15kW1/Subsystem/PLL ==
  Vgq : Inport
  Trigger : TriggerPort  VariantControl=(inherit)
  Embedded MATLAB Function : MATLAB Function  TreatAsAtomicUnit=on
  w : Outport
  wires:
  Vgq/1 -> Embedded MATLAB Function/1(Vgq)
  Embedded MATLAB Function/1(w) -> w/1

== system vnsimulink/PV15kW1/Subsystem/Subsystem ==
  vp : Inport
  vn : Inport  Port=2
  av : Inport  Port=3
  ip : Inport  Port=4
  outn : Inport  Port=5
  Enable : EnablePort
  Power Loop2 : Subsystem  TreatAsAtomicUnit=on
  Pulse Generator3 : DiscretePulseGenerator  PulseType=Time based  Period=0.0002  PulseWidth=40
  Gmax : Outport
  m : Outport  Port=2
  kii : Outport  Port=3
  ppv : Outport  Port=4
  wires:
  Power Loop2/4(m4) -> ppv/1
  Power Loop2/3(m3) -> kii/1
  outn/1 -> Power Loop2/5(outn)
  Pulse Generator3/1 -> Power Loop2/Trigger
  ip/1 -> Power Loop2/4(ip)
  av/1 -> Power Loop2/3(av)
  vn/1 -> Power Loop2/2(vn)
  vp/1 -> Power Loop2/1(vp)
  Power Loop2/2(m2) -> m/1
  Power Loop2/1(m) -> Gmax/1

== system vnsimulink/PV15kW1/Subsystem/Subsystem1 ==
  In2 : Inport
  In3 : Inport  Port=2
  Enable : EnablePort
  Out3 : Outport
  Out4 : Outport  Port=2
  wires:
  In3/1 -> Out4/1
  In2/1 -> Out3/1

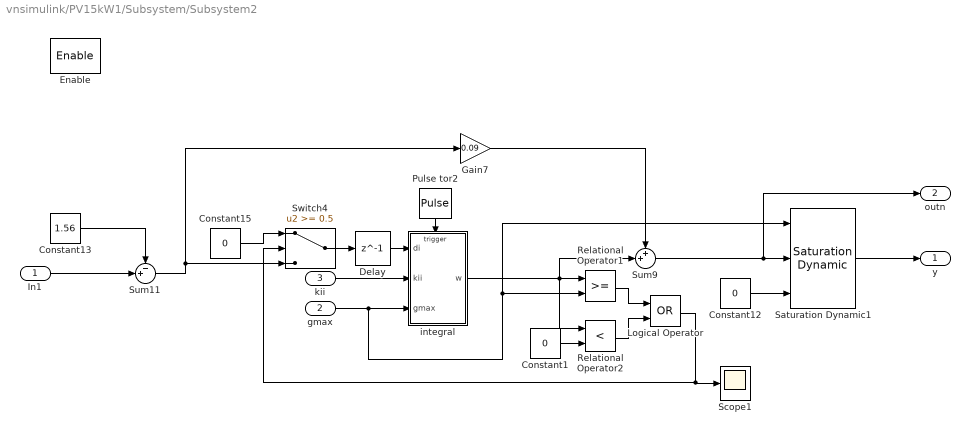
== system vnsimulink/PV15kW1/Subsystem/Subsystem2 ==
  In1 : Inport
  gmax : Inport  Port=2
  kii : Inport  Port=3
  Enable : EnablePort
  Constant1 : Constant  Value=0
  Constant12 : Constant  Value=0
  Constant13 : Constant  Value=1.56
  Constant15 : Constant  Value=0
  Delay : Delay  DelayLength=1
  Gain7 : Gain  Gain=0.09
  Logical Operator : Logic  Operator=OR  AllPortsSameDT=off  OutDataTypeStr=boolean
  Pulse tor2 : DiscretePulseGenerator  PulseType=Time based  Period=2e-4  PulseWidth=40
  Relational Operator1 : RelationalOperator  OutDataTypeStr=boolean  RndMeth=Simplest
  Relational Operator2 : RelationalOperator  Operator=<  OutDataTypeStr=boolean  RndMeth=Simplest
  Saturation Dynamic1 : simulink/Discontinuities/Saturation Dynamic  OutMin=[]  OutMax=[]  OutDataTypeStr=Inherit: Same as second input  OutDataType=fixdt(1, 16)  OutScaling=2^-10  DoSatur=off
  Scope1 : Scope
  Sum11 : Sum  Inputs=-+|
  Sum9 : Sum  Inputs=++|
  Switch4 : Switch  Threshold=0.5
  "integral " : Subsystem  TreatAsAtomicUnit=on
  y : Outport
  outn : Outport  Port=2
  wires:
  kii/1 -> "integral "/2(kii)
  Delay/1 -> "integral "/1(di)
  Pulse tor2/1 -> "integral "/Trigger
  gmax/1 -> Saturation Dynamic1/1, Relational Operator1/2, "integral "/3(gmax)
  Logical Operator/1 -> Scope1/1, Switch4/2
  Relational Operator2/1 -> Logical Operator/2
  Relational Operator1/1 -> Logical Operator/1
  Constant1/1 -> Relational Operator2/2
  Constant15/1 -> Switch4/1
  Saturation Dynamic1/1 -> y/1
  In1/1 -> Sum11/2
  Constant12/1 -> Saturation Dynamic1/3
  Gain7/1 -> Sum9/1
  "integral "/1(w) -> Relational Operator1/1, Sum9/2, Relational Operator2/1
  Switch4/1 -> Delay/1
  Sum9/1 -> Saturation Dynamic1/2, outn/1
  Sum11/1 -> Gain7/1, Switch4/3
  Constant13/1 -> Sum11/1

== system vnsimulink/PV15kW1/Subsystem/Subsystem8 ==
  In1 : Inport
  Gain : Gain
  Gain{1..2,4..5} (4 alike) : Gain  Gain=314.1593
  Gain3 : Gain  Gain=0.5
  Gain6 : Gain  Gain=0.5
  Gain7 : Gain  Gain=0.5
  Integrator{,1..3} (4 alike) : Integrator
  Sum1 : Sum  Inputs=-+-
  Sum2 : Sum  Inputs=|+-
  Sum3 : Sum  Inputs=|+-
  Out1 : Outport
  Out2 : Outport  Port=2
  wires:
  Gain7/1 -> Out2/1
  Sum1/1 -> Gain/1
  Integrator2/1 -> Sum3/2, Gain7/1
  Gain1/1 -> Integrator/1
  Sum2/1 -> Gain2/1
  Gain2/1 -> Integrator1/1
  Gain4/1 -> Integrator2/1
  Gain/1 -> Sum2/1
  Gain5/1 -> Integrator3/1
  Gain6/1 -> Out1/1
  Integrator/1 -> Sum2/2
  Integrator3/1 -> Sum1/1, Gain6/1, Gain4/1
  Gain3/1 -> Sum3/1
  Sum3/1 -> Gain5/1
  In1/1 -> Sum1/2
  Integrator1/1 -> Gain3/1, Gain1/1, Sum1/3

== system vnsimulink/PV15kW1/Subsystem/Subsystem9 ==
  In1 : Inport
  Gain : Gain
  Gain{1..2,4..5} (4 alike) : Gain  Gain=314.1593
  Gain3 : Gain  Gain=0.5
  Gain6 : Gain  Gain=0.5
  Gain7 : Gain  Gain=0.5
  Gain8 : Gain  Gain=1.815
  Gain9 : Gain  Gain=0.752
  Integrator{,1..3} (4 alike) : Integrator
  Sum1 : Sum  Inputs=-+-
  Sum2 : Sum  Inputs=|+-
  Sum3 : Sum  Inputs=|+-
  Out1 : Outport
  Out2 : Outport  Port=2
  wires:
  Integrator1/1 -> Sum1/3, Gain1/1, Gain3/1
  In1/1 -> Sum1/2
  Sum3/1 -> Gain5/1
  Gain3/1 -> Sum3/1
  Integrator3/1 -> Gain4/1, Gain6/1, Sum1/1
  Integrator/1 -> Sum2/2
  Gain6/1 -> Out1/1
  Gain5/1 -> Integrator3/1
  Gain/1 -> Sum2/1
  Gain4/1 -> Integrator2/1
  Gain2/1 -> Integrator1/1
  Sum2/1 -> Gain2/1
  Gain1/1 -> Integrator/1
  Integrator2/1 -> Gain7/1, Sum3/2
  Sum1/1 -> Gain/1
  Gain7/1 -> Out2/1

== system vnsimulink/PV15kW1/Subsystem4/Power Loop1 ==
  Vpv : Inport
  Ppv : Inport  Port=2
  Pref : Inport  Port=3
  Trigger : TriggerPort  VariantControl=(inherit)
  Embedded MATLAB Function : MATLAB Function  TreatAsAtomicUnit=on
  vpvref : Outport
  L : Outport  Port=2
  wires:
  Embedded MATLAB Function/2(l) -> L/1
  Embedded MATLAB Function/1(v) -> vpvref/1
  Ppv/1 -> Embedded MATLAB Function/2(Ppv)
  Vpv/1 -> Embedded MATLAB Function/1(Vpv)
  Pref/1 -> Embedded MATLAB Function/3(Pref)

== system vnsimulink/PV15kW2/PWM2/PWM ==
  In1 : Inport
  Bus Creator1 : BusCreator  Inputs=6
  Constant : Constant
  Demux1 : Demux  Outputs=3
  Gain : Gain  Gain=1/1
  Logical Operator : Logic  Operator=NOT  AllPortsSameDT=off  OutDataTypeStr=boolean
  Logical Operator1 : Logic  Operator=NOT  AllPortsSameDT=off  OutDataTypeStr=boolean
  Logical Operator2 : Logic  Operator=NOT  AllPortsSameDT=off  OutDataTypeStr=boolean
  Relational Operator : RelationalOperator  OutDataTypeStr=boolean  RndMeth=Nearest
  Relational Operator1 : RelationalOperator  OutDataTypeStr=boolean  RndMeth=Nearest
  Relational Operator2 : RelationalOperator  OutDataTypeStr=boolean  RndMeth=Nearest
  Repeating Sequence : simulink/Sources/Repeating Sequence  rep_seq_t=[0 1e-4 2e-4]  rep_seq_y=[0 2 0]
  Sum : Sum  Inputs=|++
  switch : Outport  PortDimensions=6
  Out1 : Outport  Port=2
  wires:
  Bus Creator1/1 -> switch/1
  Repeating Sequence/1 -> Relational Operator/2, Relational Operator1/2, Relational Operator2/2
  Constant/1 -> Sum/1
  Gain/1 -> Sum/2
  Sum/1 -> Demux1/1, Out1/1
  Demux1/1 -> Relational Operator/1
  Relational Operator/1 -> Bus Creator1/1, Logical Operator/1
  Logical Operator/1 -> Bus Creator1/2
  Demux1/2 -> Relational Operator1/1
  Relational Operator1/1 -> Bus Creator1/3, Logical Operator1/1
  Logical Operator1/1 -> Bus Creator1/4
  Demux1/3 -> Relational Operator2/1
  Relational Operator2/1 -> Bus Creator1/5, Logical Operator2/1
  Logical Operator2/1 -> Bus Creator1/6
  In1/1 -> Gain/1

== system vnsimulink/PV15kW2/Subsystem/PLL ==
  Vgq : Inport
  Trigger : TriggerPort  VariantControl=(inherit)
  Embedded MATLAB Function : MATLAB Function  TreatAsAtomicUnit=on
  w : Outport
  wires:
  Embedded MATLAB Function/1(w) -> w/1
  Vgq/1 -> Embedded MATLAB Function/1(Vgq)

== system vnsimulink/PV15kW2/Subsystem/Subsystem ==
  vp : Inport
  vn : Inport  Port=2
  av : Inport  Port=3
  ip : Inport  Port=4
  outn : Inport  Port=5
  Enable : EnablePort
  Power Loop2 : Subsystem  TreatAsAtomicUnit=on
  Pulse Generator3 : DiscretePulseGenerator  PulseType=Time based  Period=0.0002  PulseWidth=40
  Gmax : Outport
  m : Outport  Port=2
  kii : Outport  Port=3
  ppv : Outport  Port=4
  wires:
  Power Loop2/1(m) -> Gmax/1
  Power Loop2/2(m2) -> m/1
  vp/1 -> Power Loop2/1(vp)
  vn/1 -> Power Loop2/2(vn)
  av/1 -> Power Loop2/3(av)
  ip/1 -> Power Loop2/4(ip)
  Pulse Generator3/1 -> Power Loop2/Trigger
  outn/1 -> Power Loop2/5(outn)
  Power Loop2/3(m3) -> kii/1
  Power Loop2/4(m4) -> ppv/1

== system vnsimulink/PV15kW2/Subsystem/Subsystem1 ==
  In2 : Inport
  In3 : Inport  Port=2
  Enable : EnablePort
  Out3 : Outport
  Out4 : Outport  Port=2
  wires:
  In2/1 -> Out3/1
  In3/1 -> Out4/1

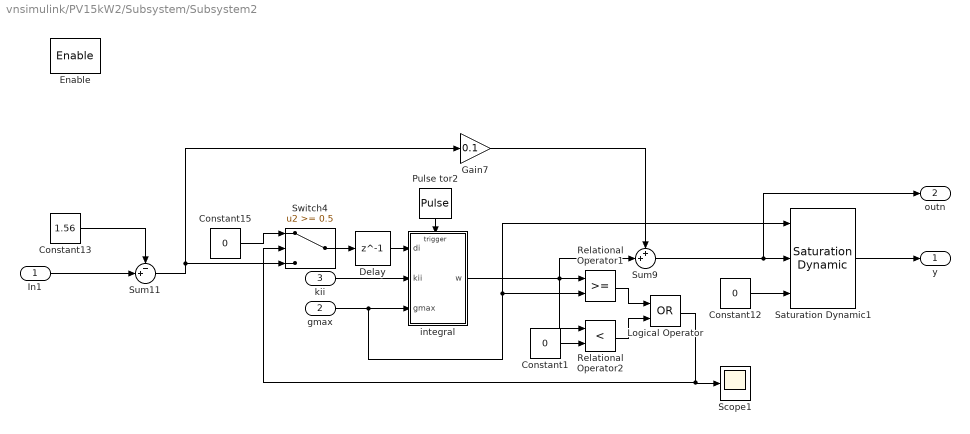
== system vnsimulink/PV15kW2/Subsystem/Subsystem2 ==
  In1 : Inport
  gmax : Inport  Port=2
  kii : Inport  Port=3
  Enable : EnablePort
  Constant1 : Constant  Value=0
  Constant12 : Constant  Value=0
  Constant13 : Constant  Value=1.56
  Constant15 : Constant  Value=0
  Delay : Delay  DelayLength=1
  Gain7 : Gain  Gain=0.1
  Logical Operator : Logic  Operator=OR  AllPortsSameDT=off  OutDataTypeStr=boolean
  Pulse tor2 : DiscretePulseGenerator  PulseType=Time based  Period=2e-4  PulseWidth=40
  Relational Operator1 : RelationalOperator  OutDataTypeStr=boolean  RndMeth=Simplest
  Relational Operator2 : RelationalOperator  Operator=<  OutDataTypeStr=boolean  RndMeth=Simplest
  Saturation Dynamic1 : simulink/Discontinuities/Saturation Dynamic  OutMin=[]  OutMax=[]  OutDataTypeStr=Inherit: Same as second input  OutDataType=fixdt(1, 16)  OutScaling=2^-10  DoSatur=off
  Scope1 : Scope
  Sum11 : Sum  Inputs=-+|
  Sum9 : Sum  Inputs=++|
  Switch4 : Switch  Threshold=0.5
  "integral " : Subsystem  TreatAsAtomicUnit=on
  y : Outport
  outn : Outport  Port=2
  wires:
  Constant13/1 -> Sum11/1
  Sum11/1 -> Switch4/3, Gain7/1
  Sum9/1 -> outn/1, Saturation Dynamic1/2
  Switch4/1 -> Delay/1
  "integral "/1(w) -> Relational Operator2/1, Sum9/2, Relational Operator1/1
  Gain7/1 -> Sum9/1
  Constant12/1 -> Saturation Dynamic1/3
  In1/1 -> Sum11/2
  Saturation Dynamic1/1 -> y/1
  Constant15/1 -> Switch4/1
  Constant1/1 -> Relational Operator2/2
  Relational Operator1/1 -> Logical Operator/1
  Relational Operator2/1 -> Logical Operator/2
  Logical Operator/1 -> Switch4/2, Scope1/1
  gmax/1 -> "integral "/3(gmax), Relational Operator1/2, Saturation Dynamic1/1
  Pulse tor2/1 -> "integral "/Trigger
  Delay/1 -> "integral "/1(di)
  kii/1 -> "integral "/2(kii)

== system vnsimulink/PV15kW2/Subsystem/Subsystem3 ==
  abc : Inport
  abc1 : Inport  Port=2
  Add2 : Sum  Inputs=+-
  Add3 : Sum
  Add4 : Sum
  Add5 : Sum  Inputs=+-
  Discrete Transfer Fcn1 : DiscreteTransferFcn  Commented=on  Numerator=[-0.9390625 1]  Denominator=[1 -0.9390625]  SampleTime=2e-4
  Discrete Transfer Fcn2 : DiscreteTransferFcn  Numerator=[-0.975177876 1]  Denominator=[1 -0.975177876]  SampleTime=8e-5
  Discrete Transfer Fcn3 : DiscreteTransferFcn  Commented=on  Numerator=[-0.93906 1]  Denominator=[1 -0.93906]  SampleTime=2e-4
  Discrete Transfer Fcn4 : DiscreteTransferFcn  Commented=on  Numerator=[-0.975177876 1]  Denominator=[1 -0.975177876]  SampleTime=8e-5
  Discrete Transfer Fcn5 : DiscreteTransferFcn  Numerator=[-0.975177876 1]  Denominator=[1 -0.975177876]  SampleTime=8e-5
  Gain{3..6} (4 alike) : Gain  Gain=0.5
  Transfer Fcn1 : TransferFcn  Commented=on  Numerator=[-1 100*pi]  Denominator=[1 100*pi]
  alpha+ : Outport
  belta+ : Outport  Port=2
  alpha- : Outport  Port=3
  belta- : Outport  Port=4
  wires:
  Discrete Transfer Fcn5/1 -> Add4/2, Add2/2  "belta’"
  Discrete Transfer Fcn2/1 -> Add5/2, Add3/1  "alpha‘"
  abc/1 -> Discrete Transfer Fcn2/1, Add4/1, Add2/1  "alpha"
  Add2/1 -> Gain3/1
  Add3/1 -> Gain4/1
  Gain6/1 -> belta-/1
  Gain5/1 -> alpha-/1
  abc1/1 -> Discrete Transfer Fcn5/1, Add3/2, Add5/1  "belta"
  Add4/1 -> Gain5/1
  Add5/1 -> Gain6/1
  Gain3/1 -> alpha+/1
  Gain4/1 -> belta+/1

== system vnsimulink/PV15kW2/Subsystem/Subsystem8 ==
  Vgq : Inport
  GIVF : Subsystem  Commented=on  TreatAsAtomicUnit=on
  Gain : Gain
  Gain{1..2,4..5} (4 alike) : Gain  Gain=314.1593
  Gain3 : Gain  Gain=0.5
  Gain6 : Gain  Gain=0.5
  Gain7 : Gain  Gain=0.5
  PID Controller{,1..3} (4 alike) : simulink/Continuous/PID Controller  Controller=I  Form=Parallel  TimeDomain=Continuous-time  UseExternalTs=off  SampleTime=2e-4  IntegratorMethod=Forward Euler  FilterMethod=Forward Euler  ControllerParametersSource=internal  P=1  I=1  D=0  UseFilter=on  N=100  TunerSelectOption=Transfer Function Based (PID Tuner App)  InitialConditionSource=internal  InitialConditionForIntegrator=0  InitialConditionForFilter=0  DifferentiatorICPrevScaledInput=0  ExternalReset=none  TrackingMode=off  Kt=1  LimitOutput=off  UpperSaturationLimit=inf  LowerSaturationLimit=-inf  LinearizeAsGain=on  AntiWindupMode=none  Kb=1  POutMin=[]  POutMax=[]  IOutMin=[]  IOutMax=[]  DOutMin=[]  DOutMax=[]  NOutMin=[]  NOutMax=[]  SumOutMin=[]  SumOutMax=[]  SaturationOutMin=[]  SaturationOutMax=[]  PParamMin=[]  PParamMax=[]  IParamMin=[]  IParamMax=[]  DParamMin=[]  DParamMax=[]  NParamMin=[]  NParamMax=[]  KbParamMin=[]  KbParamMax=[]  KtParamMin=[]  KtParamMax=[]  KbOutMin=[]  KbOutMax=[]  KtOutMin=[]  KtOutMax=[]  IntegratorOutMin=[]  IntegratorOutMax=[]  FilterOutMin=[]  FilterOutMax=[]  SumI1OutMin=[]  SumI1OutMax=[]  SumI2OutMin=[]  SumI2OutMax=[]  SumI3OutMin=[]  SumI3OutMax=[]  SumI4OutMin=[]  SumI4OutMax=[]  SumDOutMin=[]  SumDOutMax=[]  DifferentiatorOutMin=[]  DifferentiatorOutMax=[]  FilterDiffOutCoefMin=[]  FilterDiffOutCoefMax=[]  ReciprocalOutMin=[]  ReciprocalOutMax=[]  SumDenOutMin=[]  SumDenOutMax=[]  SumNumOutMin=[]  SumNumOutMax=[]  DivideOutMin=[]  DivideOutMax=[]  UdiffTsProdOutMin=[]  UdiffTsProdOutMax=[]  NTsProdOutMin=[]  NTsProdOutMax=[]  UintegralTsProdOutMin=[]  UintegralTsProdOutMax=[]  UngainTsProdOutMin=[]  UngainTsProdOutMax=[]  IntegratorContinuousStateAttributes=''  IntegratorStateMustResolveToSignalObject=off  IntegratorRTWStateStorageClass=Auto  FilterContinuousStateAttributes=''  FilterStateMustResolveToSignalObject=off  FilterRTWStateStorageClass=Auto  ParallelPVariant=Disabled  IdealPVariant=Disabled  IVariant=InternalParameters  DVariant=Disabled  IntegratorVariant=Continuous  SatVariant=Disabled  AWVariant=Passthrough  PCopyVariant=Disabled  TRVariant=Disabled  FdbkBlocksVariant=Forward  IdealPFdbkVariant=Disabled  SatFdbkVariant=Disabled  DerivativeFilterVariant=Disabled  NVariant=Disabled  NCopyVariant=Disabled_SignalSpec  FilterICVariant=Disabled  IntegratorICVariant=InternalICs  ExternalResetVariant=Disabled  TRSumVariant=Passthrough  SumFdbkVariant=Disabled  SumVariant=Passthrough_I  TsampFilterVariant=InternalTs  TsampNgainVariant=Passthrough  TsampIntegralVariant=Passthrough
  Pulse tor2 : DiscretePulseGenerator  Commented=on  PulseType=Time based  Period=2e-4  PulseWidth=40
  Sum1 : Sum  Inputs=-+-
  Sum2 : Sum  Inputs=|+-
  Sum3 : Sum  Inputs=|+-
  Out1 : Outport
  y2 : Outport  Port=2
  wires:
  PID Controller/1 -> Sum1/3, Gain1/1, Gain3/1
  Sum3/1 -> Gain5/1
  Gain3/1 -> Sum3/1
  PID Controller1/1 -> Gain4/1, Gain6/1, Sum1/1
  PID Controller3/1 -> Sum2/2
  Gain5/1 -> PID Controller1/1
  Gain/1 -> Sum2/1
  Gain4/1 -> PID Controller2/1
  Gain2/1 -> PID Controller/1
  Sum2/1 -> Gain2/1
  Gain1/1 -> PID Controller3/1
  PID Controller2/1 -> Gain7/1, Sum3/2
  Sum1/1 -> Gain/1
  Pulse tor2/1 -> GIVF/Trigger
  Vgq/1 -> Sum1/2
  Gain6/1 -> Out1/1
  Gain7/1 -> y2/1

== system vnsimulink/PV15kW2/Subsystem/Subsystem9 ==
  Vgq : Inport
  GIVF : Subsystem  Commented=on  TreatAsAtomicUnit=on
  Gain : Gain
  Gain{1..2,4..5} (4 alike) : Gain  Gain=314.1593
  Gain3 : Gain  Gain=0.5
  Gain6 : Gain  Gain=0.5
  Gain7 : Gain  Gain=0.5
  Gain8 : Gain  Gain=1.815
  Gain9 : Gain  Gain=0.752
  Integrator{,1..3} (4 alike) : Integrator
  Pulse tor2 : DiscretePulseGenerator  Commented=on  PulseType=Time based  Period=2e-4  PulseWidth=40
  Sum1 : Sum  Inputs=-+-
  Sum2 : Sum  Inputs=|+-
  Sum3 : Sum  Inputs=|+-
  Out1 : Outport
  y2 : Outport  Port=2
  wires:
  Sum1/1 -> Gain/1
  Integrator2/1 -> Sum3/2, Gain7/1
  Gain1/1 -> Integrator/1
  Sum2/1 -> Gain2/1
  Gain2/1 -> Integrator1/1
  Gain4/1 -> Integrator2/1
  Gain/1 -> Sum2/1
  Gain5/1 -> Integrator3/1
  Integrator/1 -> Sum2/2
  Integrator3/1 -> Sum1/1, Gain6/1, Gain4/1
  Gain3/1 -> Sum3/1
  Sum3/1 -> Gain5/1
  Integrator1/1 -> Gain3/1, Gain1/1, Sum1/3
  Pulse tor2/1 -> GIVF/Trigger
  Vgq/1 -> Sum1/2
  Gain6/1 -> Out1/1
  Gain7/1 -> y2/1

== system vnsimulink/PV15kW2/Subsystem4/Power Loop1 ==
  Vpv : Inport
  Ppv : Inport  Port=2
  Pref : Inport  Port=3
  Trigger : TriggerPort  VariantControl=(inherit)
  Embedded MATLAB Function : MATLAB Function  TreatAsAtomicUnit=on
  vpvref : Outport
  L : Outport  Port=2
  wires:
  Pref/1 -> Embedded MATLAB Function/3(Pref)
  Vpv/1 -> Embedded MATLAB Function/1(Vpv)
  Ppv/1 -> Embedded MATLAB Function/2(Ppv)
  Embedded MATLAB Function/1(v) -> vpvref/1
  Embedded MATLAB Function/2(l) -> L/1

== system vnsimulink/PV15kW1/Subsystem/Subsystem/Power Loop2 ==
  vp : Inport
  vn : Inport  Port=2
  av : Inport  Port=3
  ip : Inport  Port=4
  outn : Inport  Port=5
  Trigger : TriggerPort  VariantControl=(inherit)
  Pcut-sim2 : MATLAB Function  Commented=on  TreatAsAtomicUnit=on
  Pmax-sim1 : MATLAB Function  TreatAsAtomicUnit=on
  m : Outport
  m2 : Outport  Port=2
  m3 : Outport  Port=3
  m4 : Outport  Port=4
  wires:
  Pmax-sim1/4(ppv) -> m4/1
  Pmax-sim1/3(kii) -> m3/1
  Pmax-sim1/2(phi) -> m2/1
  Pmax-sim1/1(gn) -> m/1
  outn/1 -> Pmax-sim1/5(outn)
  ip/1 -> Pmax-sim1/4(ip)
  av/1 -> Pmax-sim1/3(av)
  vn/1 -> Pmax-sim1/2(vn)
  vp/1 -> Pmax-sim1/1(vp)

== system vnsimulink/PV15kW1/Subsystem/Subsystem2/integral  ==
  di : Inport
  kii : Inport  Port=2
  gmax : Inport  Port=3
  Trigger : TriggerPort  VariantControl=(inherit)
  Embedded MATLAB Function : MATLAB Function  TreatAsAtomicUnit=on
  w : Outport
  wires:
  gmax/1 -> Embedded MATLAB Function/3(gmax)
  kii/1 -> Embedded MATLAB Function/2(kii)
  di/1 -> Embedded MATLAB Function/1(di)
  Embedded MATLAB Function/1(w) -> w/1
